simulink model "SpolePlacementDesign"  (R2022b)
settings: Solver=VariableStepAuto  StartTime=0.0  StopTime=Tsim  RelTol=1e-3
libraries: cstblocks x3, simulink x1
settings Model: Creator=jprmj  LastModifiedBy=jprmj

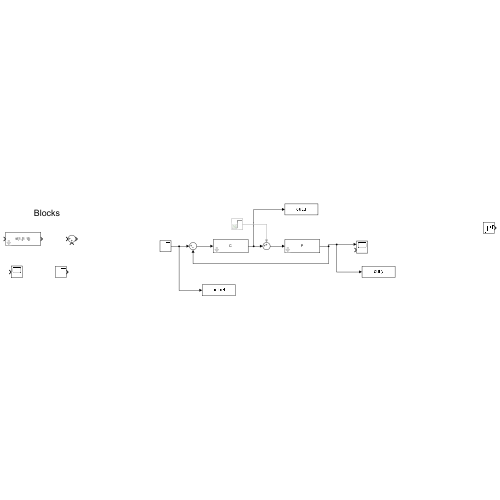
[thumbnail: Simulink's stored preview of the top-level diagram]
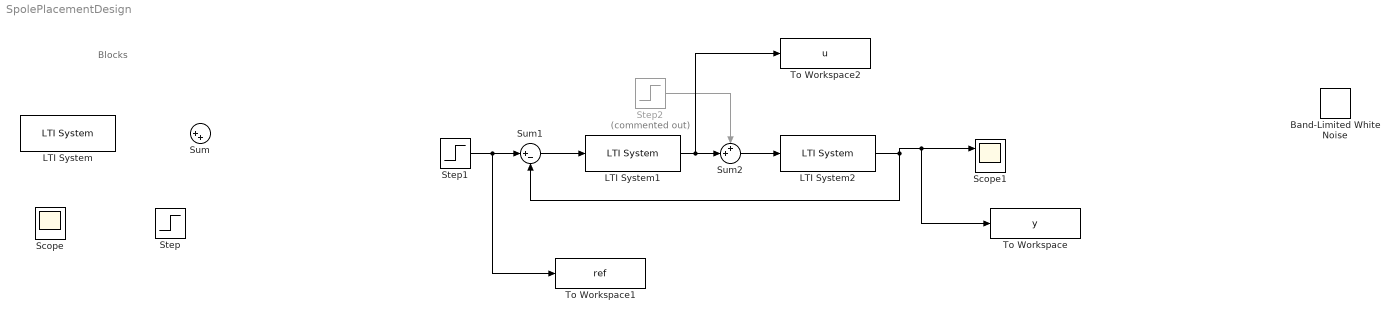
== system SpolePlacementDesign ==
  note: Blocks
  Band-Limited White Noise : simulink/Sources/Band-Limited White Noise  Cov=[0.1]  Ts=0.1  seed=[23341]
  LTI System : cstblocks/LTI System  sys=tf(1,[1 1])  IC=[]
  LTI System1 : cstblocks/LTI System  sys=C  IC=[]
  LTI System2 : cstblocks/LTI System  sys=P  IC=[]
  Scope : Scope
  Scope1 : Scope  NumInputPorts=2
  Step : Step  SampleTime=0
  Step1 : Step  SampleTime=0
  Step2 : Step  Commented=on  SampleTime=10
  Sum : Sum  Inputs=|++
  Sum1 : Sum  Inputs=|+-
  Sum2 : Sum  Inputs=++|
  To Workspace : ToWorkspace  VariableName=y  SaveFormat=Timeseries  SampleTime=-1
  To Workspace1 : ToWorkspace  VariableName=ref  SaveFormat=Timeseries  SampleTime=-1
  To Workspace2 : ToWorkspace  VariableName=u  SaveFormat=Timeseries  SampleTime=-1
  wires:
  LTI System2/1 -> To Workspace/1, Scope1/1, Sum1/2
  Step1/1 -> To Workspace1/1, Sum1/1
  Sum1/1 -> LTI System1/1
  Sum2/1 -> LTI System2/1
  Step2/1 -> Sum2/1
  LTI System1/1 -> To Workspace2/1, Sum2/2
